simulink model "Formation_no_obs"  (R2023b)
settings: Solver=FixedStepAuto  StartTime=0.0  StopTime=Sim_Time  FixedStep=dt  RelTol=1e-3
values from neighbouring files (symbols this model uses):
  delta_max = 500*pi/180    (= 8.72664625997)    [Run_Formation_no_obs.m]
  psi_r_sat = 10*pi/180    (= 0.174532925199)    [Run_Formation_no_obs.m]
  u0 = 1    [Run_Formation_no_obs.m]
  u_max = 2.5    [Run_Formation_no_obs.m]
  u_min = 0.2    [Run_Formation_no_obs.m]
  Xd = [150; 90]    [Run_Formation_no_obs.m]
  Xob = [750 800; 40 65]    [Run_Formation_no_obs.m]
libraries: slpidlib x3
settings Model: Creator=Behnaz Hadi  LastModifiedBy=ps22aae
settings SolverCC: AlgebraicLoopSolver=TrustRegion
settings DataIOCC: ReturnWorkspaceOutputs=off
settings DebuggingCC: UnconnectedInputMsg=warning  UnconnectedOutputMsg=warning  UnconnectedLineMsg=warning  ArithmeticOperatorsInVariantConditions=warning
settings ModelReferenceCC: EnableRefExpFcnMdlSchedulingChecks=on
settings SFSimCC: CustomCodeUndefinedFunction=UseInterfaceOnly
settings RTWCC: DLArmComputeVersion=19.05

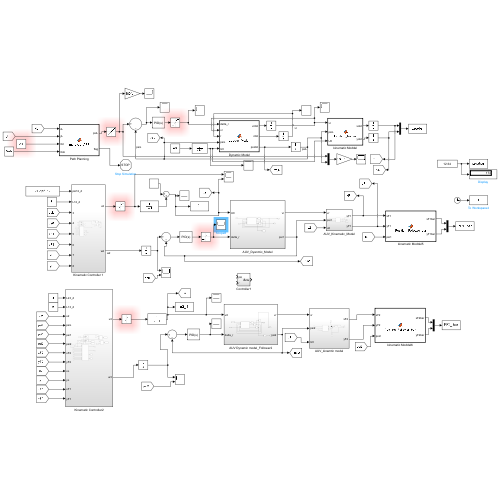
[thumbnail: Simulink's stored preview of the top-level diagram]
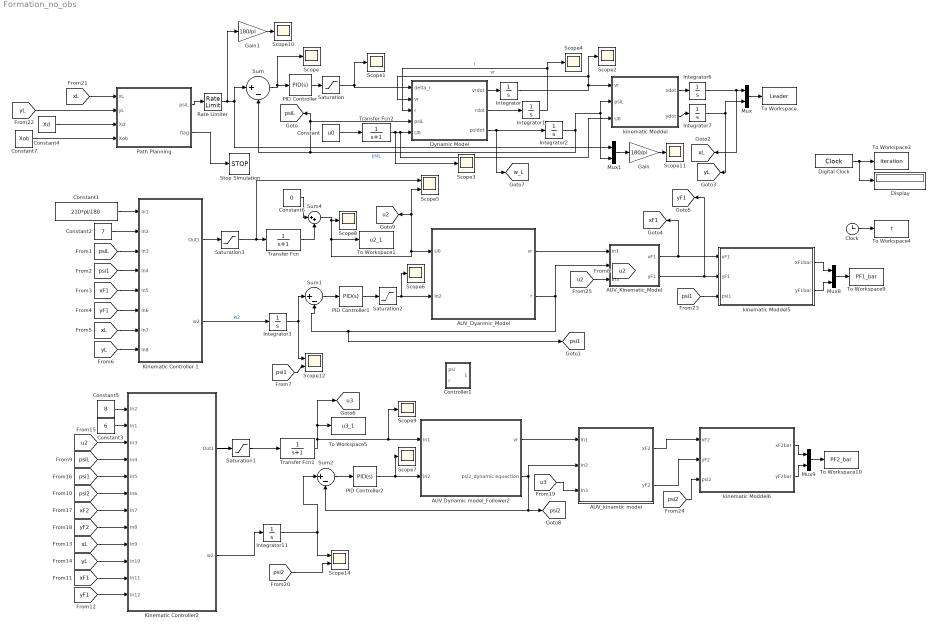
== system Formation_no_obs ==
  AUV Dynamic model_Follower2 : Subsystem
  AUV_Dyanmic_Model : Subsystem
  AUV_Kinematic_Model : Subsystem
  AUV_kinamtic model : Subsystem
  Clock : Clock
  Constant : Constant  Value=u0
  Constant1 : Constant  Value=210*pi/180
  Constant2 : Constant  Value=7
  Constant3 : Constant  Value=6
  Constant4 : Constant  Value=Xd
  Constant5 : Constant  Value=8
  Constant6 : Constant  Value=0
  Constant7 : Constant  Value=Xob
  Controller1 : Subsystem
  Digital Clock : DigitalClock
  Display : Display
  Dynamic Model : MATLAB Function  TreatAsAtomicUnit=on
  Gain : Gain  Gain=180/pi
  Gain1 : Gain  Gain=180/pi
  Integrator{,1,3,11} (4 alike) : Integrator
  Integrator2 : Integrator  InitialCondition=pi/6
  Integrator6 : Integrator  InitialCondition=6
  Integrator7 : Integrator  InitialCondition=4
  Kinematic Controller 1 : Subsystem
  Kinematic Controller2 : Subsystem
  Mux{,1,8..9} (4 alike) : Mux  Inputs=2
  PID Controller : slpidlib/PID Controller  Controller=PID  Form=Ideal  TimeDomain=Continuous-time  UseExternalTs=off  SampleTime=-1  IntegratorMethod=Forward Euler  FilterMethod=Forward Euler  ControllerParametersSource=internal  P=-4.58375331776641  I=0.348826037798542  UseKiTs=off  D=0.667672634240164  N=10.0336095861132  UseFilter=on  TunerSelectOption=Transfer Function Based (PID Tuner App)  InitialConditionSource=internal  InitialConditionForIntegrator=0  InitialConditionForFilter=0  DifferentiatorICPrevScaledInput=0  ExternalReset=none  TrackingMode=off  Kt=1  LimitOutput=off  SatLimitsSource=internal  UpperSaturationLimit=inf  LowerSaturationLimit=-inf  LinearizeAsGain=on  AntiWindupMode=none  Kb=1  LimitIntegrator=off  UpperIntegratorSaturationLimit=inf  LowerIntegratorSaturationLimit=-inf  POutMin=[]  POutMax=[]  IOutMin=[]  IOutMax=[]  DOutMin=[]  DOutMax=[]  NOutMin=[]  NOutMax=[]  SumOutMin=[]  SumOutMax=[]  SaturationOutMin=[]  SaturationOutMax=[]  PParamMin=[]  PParamMax=[]  IParamMin=[]  IParamMax=[]  DParamMin=[]  DParamMax=[]  NParamMin=[]  NParamMax=[]  KbParamMin=[]  KbParamMax=[]  KtParamMin=[]  KtParamMax=[]  KbOutMin=[]  KbOutMax=[]  KtOutMin=[]  KtOutMax=[]  IntegratorOutMin=[]  IntegratorOutMax=[]  FilterOutMin=[]  FilterOutMax=[]  SumI1OutMin=[]  SumI1OutMax=[]  SumI2OutMin=[]  SumI2OutMax=[]  SumI3OutMin=[]  SumI3OutMax=[]  SumI4OutMin=[]  SumI4OutMax=[]  SumDOutMin=[]  SumDOutMax=[]  DifferentiatorOutMin=[]  DifferentiatorOutMax=[]  FilterDiffOutCoefMin=[]  FilterDiffOutCoefMax=[]  ReciprocalOutMin=[]  ReciprocalOutMax=[]  SumDenOutMin=[]  SumDenOutMax=[]  SumNumOutMin=[]  SumNumOutMax=[]  DivideOutMin=[]  DivideOutMax=[]  UdiffTsProdOutMin=[]  UdiffTsProdOutMax=[]  NTsProdOutMin=[]  NTsProdOutMax=[]  UintegralTsProdOutMin=[]  UintegralTsProdOutMax=[]  UngainTsProdOutMin=[]  UngainTsProdOutMax=[]  ClampingZeroOutDataTypeStr=Inherit: Inherit via back propagation  ClampingZeroOutMin=[]  ClampingZeroOutMax=[]  FilterDenConstantOutDataTypeStr=Inherit: Inherit via back propagation  FilterDenConstantOutMin=[]  FilterDenConstantOutMax=[]  PCopyOutDataTypeStr=Inherit: Inherit via back propagation  PCopyOutMin=[]  PCopyOutMax=[]  NCopyOutDataTypeStr=Inherit: Inherit via back propagation  NCopyOutMin=[]  NCopyOutMax=[]  IntegratorContinuousStateAttributes=''  IntegratorStateMustResolveToSignalObject=off  IntegratorRTWStateStorageClass=Auto  FilterContinuousStateAttributes=''  FilterStateMustResolveToSignalObject=off  FilterRTWStateStorageClass=Auto  ParallelPVariant=Passthrough  IdealPVariant=InternalParameters  IVariant=InternalParameters  DVariant=InternalParameters  IntegratorVariant=Continuous  SatVariant=Disabled  AWVariant=Passthrough  PCopyVariant=Disabled  TRVariant=Disabled  FdbkBlocksVariant=Forward  IdealPFdbkVariant=Disabled  SatFdbkVariant=Disabled  DerivativeFilterVariant=ContFilter  NVariant=InternalParameters  NCopyVariant=Disabled  FilterICVariant=InternalICsFilter  IntegratorICVariant=InternalICs  ExternalResetVariant=Disabled  TRSumVariant=Passthrough  SumFdbkVariant=Disabled  SumVariant=Sum_PID  TsampFilterVariant=InternalTs  TsampNgainVariant=Passthrough  TsampIntegralVariant=Disabled_SignalSpec  ExternalSaturationOutDataTypeStr=Inherit: Same as second input
  PID Controller1 : slpidlib/PID Controller  Controller=PID  Form=Ideal  TimeDomain=Continuous-time  UseExternalTs=off  SampleTime=-1  IntegratorMethod=Forward Euler  FilterMethod=Forward Euler  ControllerParametersSource=internal  P=-4001.77706497056  I=5.16468685672513  UseKiTs=off  D=0.0301092952716466  N=1498.86057427308  UseFilter=on  TunerSelectOption=Transfer Function Based (PID Tuner App)  InitialConditionSource=internal  InitialConditionForIntegrator=0  InitialConditionForFilter=0  DifferentiatorICPrevScaledInput=0  ExternalReset=none  TrackingMode=off  Kt=1  LimitOutput=off  SatLimitsSource=internal  UpperSaturationLimit=inf  LowerSaturationLimit=-inf  LinearizeAsGain=on  AntiWindupMode=none  Kb=1  LimitIntegrator=off  UpperIntegratorSaturationLimit=inf  LowerIntegratorSaturationLimit=-inf  POutMin=[]  POutMax=[]  IOutMin=[]  IOutMax=[]  DOutMin=[]  DOutMax=[]  NOutMin=[]  NOutMax=[]  SumOutMin=[]  SumOutMax=[]  SaturationOutMin=[]  SaturationOutMax=[]  PParamMin=[]  PParamMax=[]  IParamMin=[]  IParamMax=[]  DParamMin=[]  DParamMax=[]  NParamMin=[]  NParamMax=[]  KbParamMin=[]  KbParamMax=[]  KtParamMin=[]  KtParamMax=[]  KbOutMin=[]  KbOutMax=[]  KtOutMin=[]  KtOutMax=[]  IntegratorOutMin=[]  IntegratorOutMax=[]  FilterOutMin=[]  FilterOutMax=[]  SumI1OutMin=[]  SumI1OutMax=[]  SumI2OutMin=[]  SumI2OutMax=[]  SumI3OutMin=[]  SumI3OutMax=[]  SumI4OutMin=[]  SumI4OutMax=[]  SumDOutMin=[]  SumDOutMax=[]  DifferentiatorOutMin=[]  DifferentiatorOutMax=[]  FilterDiffOutCoefMin=[]  FilterDiffOutCoefMax=[]  ReciprocalOutMin=[]  ReciprocalOutMax=[]  SumDenOutMin=[]  SumDenOutMax=[]  SumNumOutMin=[]  SumNumOutMax=[]  DivideOutMin=[]  DivideOutMax=[]  UdiffTsProdOutMin=[]  UdiffTsProdOutMax=[]  NTsProdOutMin=[]  NTsProdOutMax=[]  UintegralTsProdOutMin=[]  UintegralTsProdOutMax=[]  UngainTsProdOutMin=[]  UngainTsProdOutMax=[]  ClampingZeroOutDataTypeStr=Inherit: Inherit via back propagation  ClampingZeroOutMin=[]  ClampingZeroOutMax=[]  FilterDenConstantOutDataTypeStr=Inherit: Inherit via back propagation  FilterDenConstantOutMin=[]  FilterDenConstantOutMax=[]  PCopyOutDataTypeStr=Inherit: Inherit via back propagation  PCopyOutMin=[]  PCopyOutMax=[]  NCopyOutDataTypeStr=Inherit: Inherit via back propagation  NCopyOutMin=[]  NCopyOutMax=[]  IntegratorContinuousStateAttributes=''  IntegratorStateMustResolveToSignalObject=off  IntegratorRTWStateStorageClass=Auto  FilterContinuousStateAttributes=''  FilterStateMustResolveToSignalObject=off  FilterRTWStateStorageClass=Auto  ParallelPVariant=Passthrough  IdealPVariant=InternalParameters  IVariant=InternalParameters  DVariant=InternalParameters  IntegratorVariant=Continuous  SatVariant=Disabled  AWVariant=Passthrough  PCopyVariant=Disabled  TRVariant=Disabled  FdbkBlocksVariant=Forward  IdealPFdbkVariant=Disabled  SatFdbkVariant=Disabled  DerivativeFilterVariant=ContFilter  NVariant=InternalParameters  NCopyVariant=Disabled  FilterICVariant=InternalICsFilter  IntegratorICVariant=InternalICs  ExternalResetVariant=Disabled  TRSumVariant=Passthrough  SumFdbkVariant=Disabled  SumVariant=Sum_PID  TsampFilterVariant=InternalTs  TsampNgainVariant=Passthrough  TsampIntegralVariant=Disabled_SignalSpec  ExternalSaturationOutDataTypeStr=Inherit: Same as second input
  PID Controller2 : slpidlib/PID Controller  Controller=PID  Form=Ideal  TimeDomain=Continuous-time  UseExternalTs=off  SampleTime=-1  IntegratorMethod=Forward Euler  FilterMethod=Forward Euler  ControllerParametersSource=internal  P=-22  I=0  UseKiTs=off  D=0.4  N=68.9458315113197  UseFilter=on  TunerSelectOption=Transfer Function Based (PID Tuner App)  InitialConditionSource=internal  InitialConditionForIntegrator=0  InitialConditionForFilter=0  DifferentiatorICPrevScaledInput=0  ExternalReset=none  TrackingMode=off  Kt=1  LimitOutput=off  SatLimitsSource=internal  UpperSaturationLimit=inf  LowerSaturationLimit=-inf  LinearizeAsGain=on  AntiWindupMode=none  Kb=1  LimitIntegrator=off  UpperIntegratorSaturationLimit=inf  LowerIntegratorSaturationLimit=-inf  POutMin=[]  POutMax=[]  IOutMin=[]  IOutMax=[]  DOutMin=[]  DOutMax=[]  NOutMin=[]  NOutMax=[]  SumOutMin=[]  SumOutMax=[]  SaturationOutMin=[]  SaturationOutMax=[]  PParamMin=[]  PParamMax=[]  IParamMin=[]  IParamMax=[]  DParamMin=[]  DParamMax=[]  NParamMin=[]  NParamMax=[]  KbParamMin=[]  KbParamMax=[]  KtParamMin=[]  KtParamMax=[]  KbOutMin=[]  KbOutMax=[]  KtOutMin=[]  KtOutMax=[]  IntegratorOutMin=[]  IntegratorOutMax=[]  FilterOutMin=[]  FilterOutMax=[]  SumI1OutMin=[]  SumI1OutMax=[]  SumI2OutMin=[]  SumI2OutMax=[]  SumI3OutMin=[]  SumI3OutMax=[]  SumI4OutMin=[]  SumI4OutMax=[]  SumDOutMin=[]  SumDOutMax=[]  DifferentiatorOutMin=[]  DifferentiatorOutMax=[]  FilterDiffOutCoefMin=[]  FilterDiffOutCoefMax=[]  ReciprocalOutMin=[]  ReciprocalOutMax=[]  SumDenOutMin=[]  SumDenOutMax=[]  SumNumOutMin=[]  SumNumOutMax=[]  DivideOutMin=[]  DivideOutMax=[]  UdiffTsProdOutMin=[]  UdiffTsProdOutMax=[]  NTsProdOutMin=[]  NTsProdOutMax=[]  UintegralTsProdOutMin=[]  UintegralTsProdOutMax=[]  UngainTsProdOutMin=[]  UngainTsProdOutMax=[]  ClampingZeroOutDataTypeStr=Inherit: Inherit via back propagation  ClampingZeroOutMin=[]  ClampingZeroOutMax=[]  FilterDenConstantOutDataTypeStr=Inherit: Inherit via back propagation  FilterDenConstantOutMin=[]  FilterDenConstantOutMax=[]  PCopyOutDataTypeStr=Inherit: Inherit via back propagation  PCopyOutMin=[]  PCopyOutMax=[]  NCopyOutDataTypeStr=Inherit: Inherit via back propagation  NCopyOutMin=[]  NCopyOutMax=[]  IntegratorContinuousStateAttributes=''  IntegratorStateMustResolveToSignalObject=off  IntegratorRTWStateStorageClass=Auto  FilterContinuousStateAttributes=''  FilterStateMustResolveToSignalObject=off  FilterRTWStateStorageClass=Auto  ParallelPVariant=Passthrough  IdealPVariant=InternalParameters  IVariant=InternalParameters  DVariant=InternalParameters  IntegratorVariant=Continuous  SatVariant=Disabled  AWVariant=Passthrough  PCopyVariant=Disabled  TRVariant=Disabled  FdbkBlocksVariant=Forward  IdealPFdbkVariant=Disabled  SatFdbkVariant=Disabled  DerivativeFilterVariant=ContFilter  NVariant=InternalParameters  NCopyVariant=Disabled  FilterICVariant=InternalICsFilter  IntegratorICVariant=InternalICs  ExternalResetVariant=Disabled  TRSumVariant=Passthrough  SumFdbkVariant=Disabled  SumVariant=Sum_PID  TsampFilterVariant=InternalTs  TsampNgainVariant=Passthrough  TsampIntegralVariant=Disabled_SignalSpec  ExternalSaturationOutDataTypeStr=Inherit: Same as second input
  Path Planning : MATLAB Function  TreatAsAtomicUnit=on
  Rate Limiter : RateLimiter  RisingSlewLimit=psi_r_sat  FallingSlewLimit=-psi_r_sat  SampleTimeMode=inherited
  Saturation : Saturate  UpperLimit=delta_max  LowerLimit=-delta_max
  Saturation1 : Saturate  UpperLimit=u_max  LowerLimit=u_min
  Saturation2 : Saturate  UpperLimit=delta_max  LowerLimit=-delta_max
  Saturation3 : Saturate  UpperLimit=u_max  LowerLimit=u_min
  Scope{,1..4,6..11} (11 alike) : Scope
  Scope12 : Scope  NumInputPorts=2
  Scope14 : Scope  NumInputPorts=2
  Scope5 : Scope  NumInputPorts=2
  Stop Simulation : Stop
  Sum : Sum  Inputs=|+-
  Sum1 : Sum  Inputs=|+-
  Sum2 : Sum  Inputs=|+-
  Sum4 : Sum  Inputs=|++
  To Workspace : ToWorkspace  VariableName=Leader  SampleTime=-1
  To Workspace1 : ToWorkspace  VariableName=u2_1  SampleTime=-1
  To Workspace10 : ToWorkspace  VariableName=PF2_bar  SampleTime=-1
  To Workspace3 : ToWorkspace  VariableName=iteration  SampleTime=-1
  To Workspace4 : ToWorkspace  VariableName=t  SampleTime=-1
  To Workspace5 : ToWorkspace  VariableName=u3_1  SampleTime=-1
  To Workspace9 : ToWorkspace  VariableName=PF1_bar  SampleTime=-1
  Transfer Fcn : TransferFcn  Denominator=[1 1]
  Transfer Fcn1 : TransferFcn  Denominator=[1 1]
  Transfer Fcn2 : TransferFcn  Denominator=[1 1]
  kinematic Moddel : MATLAB Function  TreatAsAtomicUnit=on
  kinematic Moddel5 : MATLAB Function  TreatAsAtomicUnit=on
  kinematic Moddel6 : MATLAB Function  TreatAsAtomicUnit=on
  tag scope: psi1=global, psi2=global, psiL=global, u2=global, u3=global, w_L=global, xF1=global, xL=global, yF1=global, yL=global
  wires:
  [xL] -> Path Planning/1(xL)
  [yL] -> Path Planning/2(yL)
  Path Planning/2(flag) -> Stop Simulation/1
  Path Planning/1(psiL) -> Rate Limiter/1
  kinematic Moddel/1(xdot) -> Integrator6/1
  Integrator6/1 -> [xL], Mux/1
  kinematic Moddel/2(ydot) -> Integrator7/1
  Mux1/1 -> Gain/1
  Integrator1/1 -> Scope4/1, Dynamic Model/3(r)  "r"
  Dynamic Model/1(vrdot) -> Integrator/1
  Saturation/1 -> Dynamic Model/1(delta_r), Scope1/1
  Dynamic Model/3(psidot) -> Integrator2/1, [w_L]
  Integrator2/1 -> Mux1/2, kinematic Moddel/2(psiL), Dynamic Model/4(psiL), [psiL], Sum/2  "psiL"
  Sum/1 -> PID Controller/1, Scope/1
  Integrator7/1 -> [yL], Mux/2
  Integrator/1 -> Dynamic Model/2(vr), Scope2/1, kinematic Moddel/1(vr)  "vr"
  Mux/1 -> To Workspace/1
  Dynamic Model/2(rdot) -> Integrator1/1
  Clock/1 -> To Workspace4/1
  Digital Clock/1 -> Display/1, To Workspace3/1
  Sum1/1 -> PID Controller1/1
  Sum2/1 -> PID Controller2/1
  kinematic Moddel5/1(xF1bar) -> Mux8/1
  kinematic Moddel5/2(yF1bar) -> Mux8/2
  Mux8/1 -> To Workspace9/1
  kinematic Moddel6/2(yF2bar) -> Mux9/2
  kinematic Moddel6/1(xF2bar) -> Mux9/1
  Mux9/1 -> To Workspace10/1
  [psi2] -> kinematic Moddel6/3(psi2)
  Kinematic Controller 1/2(w2) -> Integrator3/1  "w2"
  Constant1/1 -> Kinematic Controller 1/1(In1)
  Constant2/1 -> Kinematic Controller 1/2(In2)
  [psiL] -> Kinematic Controller 1/3(In3)
  [psi1] -> Kinematic Controller 1/4(In4)
  [xF1] -> Kinematic Controller 1/5(In5)
  [yF1] -> Kinematic Controller 1/6(In6)
  [xL] -> Kinematic Controller 1/7(In7)
  [yL] -> Kinematic Controller 1/8(In8)
  AUV_Dyanmic_Model/2(r) -> AUV_Kinematic_Model/2(In2), Sum1/2, [psi1]
  Kinematic Controller 1/1(Out1) -> Saturation3/1
  [psi1] -> Scope12/2
  AUV_Dyanmic_Model/1(vr) -> AUV_Kinematic_Model/1(In1)
  [u2] -> AUV_Kinematic_Model/3(In3)
  AUV_Kinematic_Model/1(xF1) -> [xF1], kinematic Moddel5/1(xF1)
  AUV_Kinematic_Model/2(yF1) -> [yF1], kinematic Moddel5/2(yF1)
  [psi1] -> kinematic Moddel5/3(psi1)
  Kinematic Controller2/2(w2) -> Integrator11/1
  Constant3/1 -> Kinematic Controller2/2(In1)
  [u2] -> Kinematic Controller2/3(In3)
  [psiL] -> Kinematic Controller2/4(In4)
  [psi1] -> Kinematic Controller2/5(In5)
  [psi2] -> Kinematic Controller2/6(In6)
  [xF2] -> Kinematic Controller2/7(In7)
  [yF2] -> Kinematic Controller2/8(In8)
  [xL] -> Kinematic Controller2/9(In9)
  [yL] -> Kinematic Controller2/10(In10)
  [xF1] -> Kinematic Controller2/11(In11)
  [yF1] -> Kinematic Controller2/12(In12)
  Constant5/1 -> Kinematic Controller2/1(In2)
  AUV Dynamic model_Follower2/2(psi2_dynamic equaction) -> AUV_kinamtic model/2(In2), [psi2], Sum2/2
  Kinematic Controller2/1(Out1) -> Saturation1/1
  [psi2] -> Scope14/2
  AUV Dynamic model_Follower2/1(vr) -> AUV_kinamtic model/1(In1)
  [u3] -> AUV_kinamtic model/3(In3)
  AUV_kinamtic model/1(xF2) -> kinematic Moddel6/1(xF2)
  AUV_kinamtic model/2(yF2) -> kinematic Moddel6/2(yF2)
  Integrator11/1 -> Scope14/1, Sum2/1
  Integrator3/1 -> Scope12/1, Sum1/1
  Sum4/1 -> Scope5/2, [u2], AUV_Dyanmic_Model/1(U0), To Workspace1/1, Scope8/1
  Transfer Fcn1/1 -> [u3], To Workspace5/1, Scope9/1, AUV Dynamic model_Follower2/1(In1)
  PID Controller2/1 -> AUV Dynamic model_Follower2/2(In2), Scope7/1
  PID Controller/1 -> Saturation/1
  Rate Limiter/1 -> Gain1/1, Sum/1, Mux1/1
  PID Controller1/1 -> Saturation2/1
  Gain/1 -> Scope11/1
  Gain1/1 -> Scope10/1
  Constant/1 -> Transfer Fcn2/1
  Saturation2/1 -> Scope6/1, AUV_Dyanmic_Model/2(In2)
  Transfer Fcn/1 -> Sum4/2
  Constant6/1 -> Sum4/1
  Constant4/1 -> Path Planning/3(Xd)
  Constant7/1 -> Path Planning/4(Xob)
  Saturation1/1 -> Transfer Fcn1/1
  Saturation3/1 -> Transfer Fcn/1, Scope5/1
  Transfer Fcn2/1 -> Scope3/1, kinematic Moddel/3(U0), Dynamic Model/5(U0)

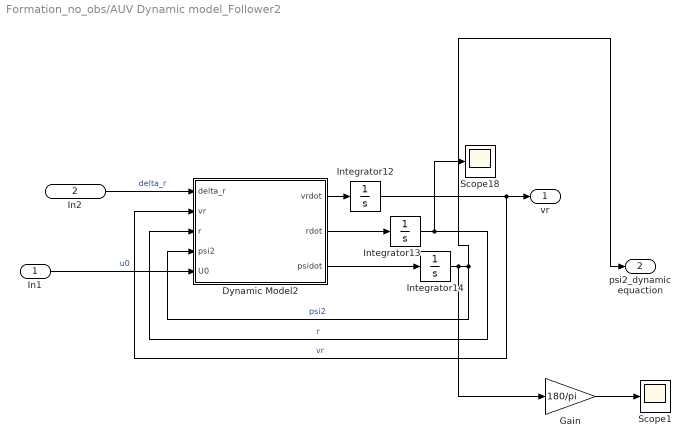
== system Formation_no_obs/AUV Dynamic model_Follower2 ==
  In1 : Inport
  In2 : Inport  Port=2
  Dynamic Model2 : MATLAB Function  TreatAsAtomicUnit=on
  Gain : Gain  Gain=180/pi
  Integrator12 : Integrator
  Integrator13 : Integrator
  Integrator14 : Integrator  InitialCondition=pi/6
  Scope1 : Scope
  Scope18 : Scope
  vr : Outport  VectorParamsAs1DForOutWhenUnconnected=off
  psi2_dynamic equaction : Outport  Port=2  VectorParamsAs1DForOutWhenUnconnected=off
  wires:
  In1/1 -> Dynamic Model2/5(U0)  "u0"
  Dynamic Model2/2(rdot) -> Integrator13/1
  Integrator13/1 -> Scope18/1, Dynamic Model2/3(r)  "r"
  In2/1 -> Dynamic Model2/1(delta_r)  "delta_r"
  Integrator12/1 -> vr/1, Dynamic Model2/2(vr)  "vr"
  Dynamic Model2/3(psidot) -> Integrator14/1
  Dynamic Model2/1(vrdot) -> Integrator12/1
  Integrator14/1 -> Gain/1, psi2_dynamic equaction/1, Dynamic Model2/4(psi2)  "psi2"
  Gain/1 -> Scope1/1

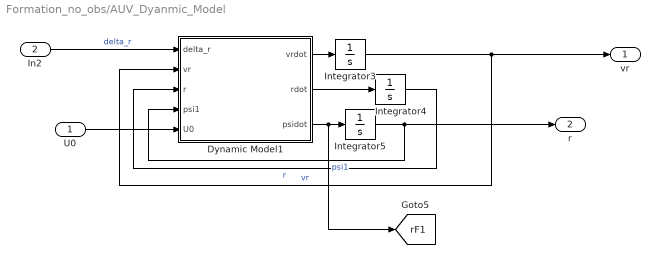
== system Formation_no_obs/AUV_Dyanmic_Model ==
  U0 : Inport
  In2 : Inport  Port=2
  Dynamic Model1 : MATLAB Function  TreatAsAtomicUnit=on
  Integrator3 : Integrator
  Integrator4 : Integrator
  Integrator5 : Integrator
  vr : Outport  VectorParamsAs1DForOutWhenUnconnected=off
  r : Outport  Port=2  VectorParamsAs1DForOutWhenUnconnected=off
  tag scope: rF1=global
  wires:
  Integrator4/1 -> Dynamic Model1/3(r)  "r"
  Dynamic Model1/1(vrdot) -> Integrator3/1
  Dynamic Model1/2(rdot) -> Integrator4/1
  Dynamic Model1/3(psidot) -> [rF1], Integrator5/1
  U0/1 -> Dynamic Model1/5(U0)
  Integrator3/1 -> vr/1, Dynamic Model1/2(vr)  "vr"
  Integrator5/1 -> Dynamic Model1/4(psi1), r/1  "psi1"
  In2/1 -> Dynamic Model1/1(delta_r)  "delta_r"

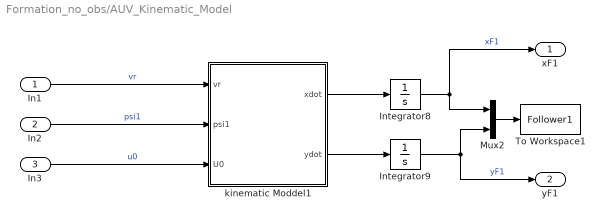
== system Formation_no_obs/AUV_Kinematic_Model ==
  In1 : Inport
  In2 : Inport  Port=2
  In3 : Inport  Port=3
  Integrator8 : Integrator  InitialCondition=7
  Integrator9 : Integrator  InitialCondition=2
  Mux2 : Mux  Inputs=2
  To Workspace1 : ToWorkspace  VariableName=Follower1  SampleTime=-1
  kinematic Moddel1 : MATLAB Function  TreatAsAtomicUnit=on
  xF1 : Outport  VectorParamsAs1DForOutWhenUnconnected=off
  yF1 : Outport  Port=2  VectorParamsAs1DForOutWhenUnconnected=off
  wires:
  kinematic Moddel1/2(ydot) -> Integrator9/1
  kinematic Moddel1/1(xdot) -> Integrator8/1
  Mux2/1 -> To Workspace1/1
  Integrator9/1 -> yF1/1, Mux2/2  "yF1"
  Integrator8/1 -> Mux2/1, xF1/1  "xF1"
  In1/1 -> kinematic Moddel1/1(vr)  "vr"
  In2/1 -> kinematic Moddel1/2(psi1)  "psi1"
  In3/1 -> kinematic Moddel1/3(U0)  "u0"

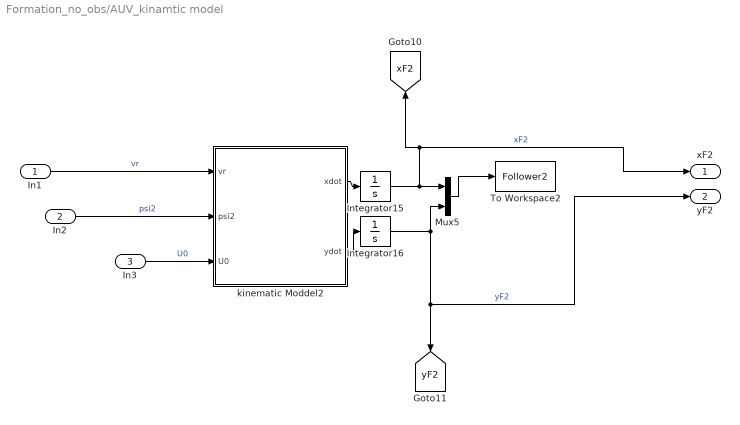
== system Formation_no_obs/AUV_kinamtic model ==
  In1 : Inport
  In2 : Inport  Port=2
  In3 : Inport  Port=3
  Integrator15 : Integrator  InitialCondition=2
  Integrator16 : Integrator  InitialCondition=1
  Mux5 : Mux  Inputs=2
  To Workspace2 : ToWorkspace  VariableName=Follower2  SampleTime=-1
  kinematic Moddel2 : MATLAB Function  TreatAsAtomicUnit=on
  xF2 : Outport  VectorParamsAs1DForOutWhenUnconnected=off
  yF2 : Outport  Port=2  VectorParamsAs1DForOutWhenUnconnected=off
  tag scope: xF2=global, yF2=global
  wires:
  Integrator15/1 -> xF2/1, [xF2], Mux5/1  "xF2"
  Integrator16/1 -> Mux5/2, yF2/1, [yF2]  "yF2"
  kinematic Moddel2/2(ydot) -> Integrator16/1
  In1/1 -> kinematic Moddel2/1(vr)  "vr"
  kinematic Moddel2/1(xdot) -> Integrator15/1
  Mux5/1 -> To Workspace2/1
  In3/1 -> kinematic Moddel2/3(U0)  "U0"
  In2/1 -> kinematic Moddel2/2(psi2)  "psi2"

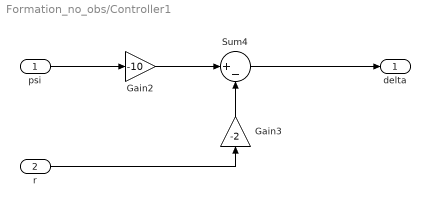
== system Formation_no_obs/Controller1 ==
  psi : Inport
  r : Inport  Port=2
  Gain2 : Gain  Gain=-10
  Gain3 : Gain  Gain=-2
  Sum4 : Sum  Inputs=|+-
  delta : Outport
  wires:
  Gain2/1 -> Sum4/1
  Gain3/1 -> Sum4/2
  psi/1 -> Gain2/1
  Sum4/1 -> delta/1
  r/1 -> Gain3/1

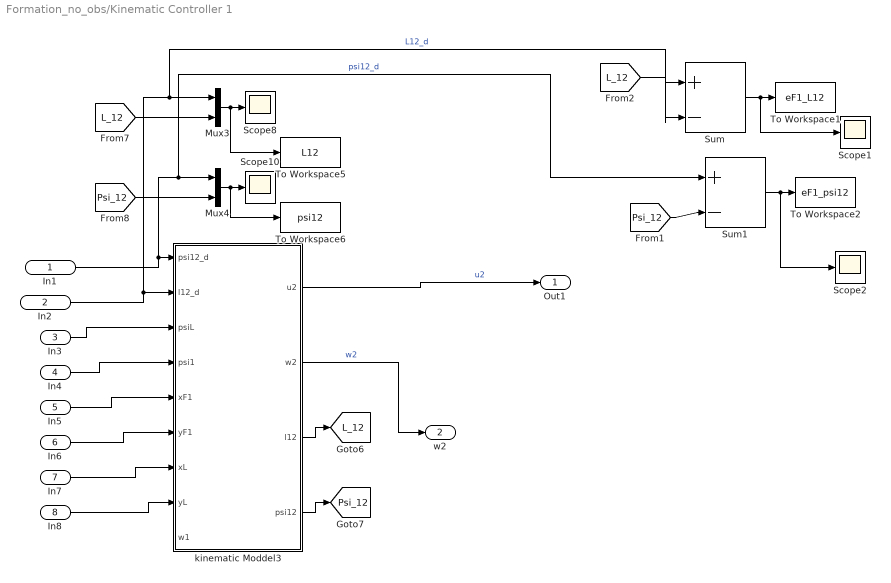
== system Formation_no_obs/Kinematic Controller 1 ==
  In1 : Inport
  In2 : Inport  Port=2
  In3 : Inport  Port=3
  In4 : Inport  Port=4
  In5 : Inport  Port=5
  In6 : Inport  Port=6
  In7 : Inport  Port=7
  In8 : Inport  Port=8
  Mux3 : Mux  Inputs=2
  Mux4 : Mux  Inputs=2
  Scope{1..2,8,10} (4 alike) : Scope
  Sum : Sum  Inputs=+|-
  Sum1 : Sum  Inputs=+|-
  To Workspace1 : ToWorkspace  VariableName=eF1_L12  SampleTime=-1
  To Workspace2 : ToWorkspace  VariableName=eF1_psi12  SampleTime=-1
  To Workspace5 : ToWorkspace  VariableName=L12  SampleTime=-1
  To Workspace6 : ToWorkspace  VariableName=psi12  SampleTime=-1
  kinematic Moddel3 : MATLAB Function  TreatAsAtomicUnit=on
  Out1 : Outport  VectorParamsAs1DForOutWhenUnconnected=off
  w2 : Outport  Port=2  VectorParamsAs1DForOutWhenUnconnected=off
  tag scope: L_12=global, Psi_12=global
  wires:
  Mux3/1 -> To Workspace5/1, Scope8/1
  [Psi_12] -> Mux4/2
  [L_12] -> Mux3/2
  In8/1 -> kinematic Moddel3/8(yL)
  Mux4/1 -> To Workspace6/1, Scope10/1
  kinematic Moddel3/4(psi12) -> [Psi_12]
  In3/1 -> kinematic Moddel3/3(psiL)
  kinematic Moddel3/3(l12) -> [L_12]
  kinematic Moddel3/2(w2) -> w2/1  "w2"
  In4/1 -> kinematic Moddel3/4(psi1)
  In5/1 -> kinematic Moddel3/5(xF1)
  In6/1 -> kinematic Moddel3/6(yF1)
  In7/1 -> kinematic Moddel3/7(xL)
  kinematic Moddel3/1(u2) -> Out1/1  "u2"
  In2/1 -> Sum/1, Mux3/1, kinematic Moddel3/2(l12_d)  "L12_d"
  In1/1 -> Sum1/1, Mux4/1, kinematic Moddel3/1(psi12_d)  "psi12_d"
  [Psi_12] -> Sum1/2
  Sum1/1 -> Scope2/1, To Workspace2/1
  Sum/1 -> Scope1/1, To Workspace1/1
  [L_12] -> Sum/2

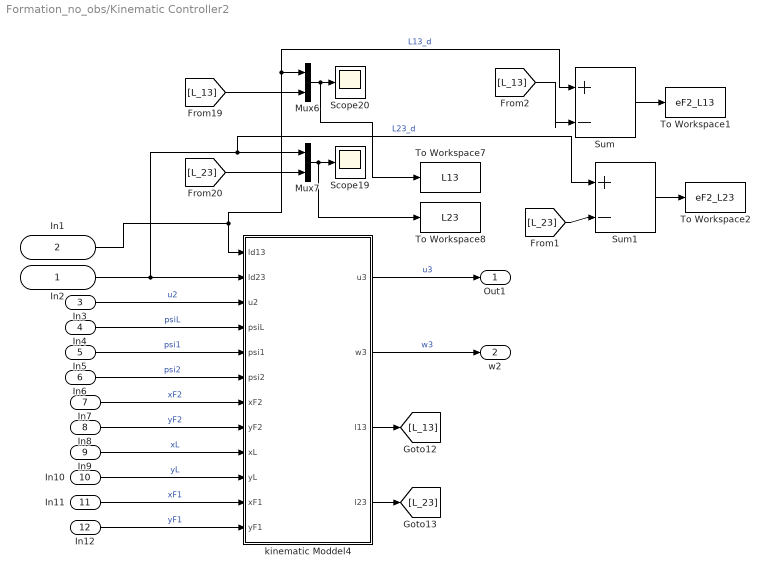
== system Formation_no_obs/Kinematic Controller2 ==
  In2 : Inport
  In1 : Inport  Port=2
  In3 : Inport  Port=3
  In4 : Inport  Port=4
  In5 : Inport  Port=5
  In6 : Inport  Port=6
  In7 : Inport  Port=7
  In8 : Inport  Port=8
  In9 : Inport  Port=9
  In10 : Inport  Port=10
  In11 : Inport  Port=11
  In12 : Inport  Port=12
  Mux6 : Mux  Inputs=2
  Mux7 : Mux  Inputs=2
  Scope19 : Scope
  Scope20 : Scope
  Sum : Sum  Inputs=+|-
  Sum1 : Sum  Inputs=+|-
  To Workspace1 : ToWorkspace  VariableName=eF2_L13  SampleTime=-1
  To Workspace2 : ToWorkspace  VariableName=eF2_L23  SampleTime=-1
  To Workspace7 : ToWorkspace  VariableName=L13  SampleTime=-1
  To Workspace8 : ToWorkspace  VariableName=L23  SampleTime=-1
  kinematic Moddel4 : MATLAB Function  TreatAsAtomicUnit=on
  Out1 : Outport  VectorParamsAs1DForOutWhenUnconnected=off
  w2 : Outport  Port=2  VectorParamsAs1DForOutWhenUnconnected=off
  wires:
  In8/1 -> kinematic Moddel4/8(yF2)  "yF2"
  In6/1 -> kinematic Moddel4/6(psi2)  "psi2"
  kinematic Moddel4/4(l23) -> [L_23]
  In12/1 -> kinematic Moddel4/12(yF1)  "yF1"
  In1/1 -> kinematic Moddel4/1(ld13), Sum/1, Mux6/1  "L13_d"
  [L_23] -> Mux7/2
  Mux7/1 -> To Workspace8/1, Scope19/1
  Mux6/1 -> To Workspace7/1, Scope20/1
  [L_13] -> Mux6/2
  kinematic Moddel4/3(l13) -> [L_13]
  In4/1 -> kinematic Moddel4/4(psiL)  "psiL"
  In10/1 -> kinematic Moddel4/10(yL)  "yL"
  kinematic Moddel4/1(u3) -> Out1/1  "u3"
  In7/1 -> kinematic Moddel4/7(xF2)  "xF2"
  In3/1 -> kinematic Moddel4/3(u2)  "u2"
  kinematic Moddel4/2(w3) -> w2/1  "w3"
  In11/1 -> kinematic Moddel4/11(xF1)  "xF1"
  In5/1 -> kinematic Moddel4/5(psi1)  "psi1"
  In9/1 -> kinematic Moddel4/9(xL)  "xL"
  [L_13] -> Sum/2
  Sum/1 -> To Workspace1/1
  Sum1/1 -> To Workspace2/1
  In2/1 -> kinematic Moddel4/2(ld23), Mux7/1, Sum1/1  "L23_d"
  [L_23] -> Sum1/2

== matlab function Formation_no_obs/AUV_kinamtic model/kinematic Moddel2 ==
  data: vr input; psi2 input; xdot output; ydot output; U0 input
function [xdot,ydot] = Position_Follower(vr,psi2,U0)
% global U0
% U0 = 1.3;
% Ucx =0.2; Ucy =0.2; 
Ucx =0.0; Ucy =0.0; 


% x_dot = U0*cos(sa) - vr*sin(sa)+Ucx;
% y_dot = U0*sin(sa) + vr*cos(sa)+Ucy;
xdot  = U0*cos(psi2) - vr*sin(psi2)+ Ucx ;  %x_dot
ydot  = U0*sin(psi2) + vr*cos(psi2)+ Ucy ;  %y_dot

end

== matlab function Formation_no_obs/Kinematic Controller2/kinematic Moddel4 ==
  data: ld13 input; ld23 input; u2 input; psiL input; psi1 input; psi2 input; u3 output; w3 output; xF2 input; yF2 input; xL input; yL input; xF1 input; yF1 input; l13 output; l23 output
function [u3, w3, l13, l23] = Desai_Controller_TwoNeighbors(ld13, ld23, u2, psiL, psi1, psi2, xF2, yF2, xL, yL, xF1, yF1)
    % Parameters
    u1 = 1.0; d = 0.16;
    alpha1 = 0.2; alpha2 = 0.2;

    % Virtual target point for agent 3 (distance d ahead of follower 2)
    x3b = xF2 + d * cos(psi2);
    y3b = yF2 + d * sin(psi2);

    % psi13: angle from agent L to 3bar
    atan13 = atan2(y3b - yL, x3b - xL);
    if atan13 < 0
        psi13 = 2 * pi + atan13 - psiL;
    else
        psi13 = atan13 - psiL;
    end

    % psi23: angle from agent 1 to 3bar
    atan23 = atan2(y3b - yF1, x3b - xF1);
    if atan23 < 0
        psi23 = 2 * pi + atan23 - psi1;
    else
        psi23 = atan23 - psi1;
    end

    % Inter-agent distances
    l13 = sqrt((xL - x3b)^2 + (yL - y3b)^2);
    l23 = sqrt((xF1 - x3b)^2 + (yF1 - y3b)^2);

    % Heading errors
    gamma1 = psiL + psi13 - psi2;
    gamma2 = psi1 + psi23 - psi2;

    % Wrap angles
    gamma1 = atan2(sin(gamma1), cos(gamma1));
    gamma2 = atan2(sin(gamma2), cos(gamma2));

    % Angular velocity w3
    w3 = (1 / (d * sin(gamma1 - gamma2))) * ...
         ( alpha1 * (ld13 - l13) * cos(gamma2) + u1 * cos(psi13) * cos(gamma2) ...
         - alpha2 * (ld23 - l23) * cos(gamma1) - u2 * cos(psi23) * cos(gamma1) );

    % Linear velocity u3
    u3 = (alpha1 * (ld13 - l13) + u1 * cos(psi13) - d * w3 * sin(gamma1)) / cos(gamma1);
end

== matlab function Formation_no_obs/Path Planning ==
  data: xL input; psiL output; yL input; flag output; Xd input; Xob input
%%%%%%%%%%%%%%% The Basid Method in the book, uncomment if needed %%%%%%%%%
%%%%%%%%%%%%%%%%%%%%%%%%%%%%%%%%%%%%%%%%%%%%%%%%%%%%%%%%%%%%%%%%%%%%%%%%%%%
% function [psiL, flag] = improved_APF(xL, yL, Xd, Xob)
%     % Parameters
%     K_att = 1.0;       % Attractive gain
%     K_rep = 100;         % Repulsive gain
%     rho_0 = 15;        % Repulsion influence range
%     R = 8;             % Obstacle radius
%     flag = 0;          % Goal reached flag
% 
%     % Positions
%     r = [xL; yL];      % Current position
%     rd = Xd;           % Goal position
% 
%     % Attractive force
%     Fatt = -K_att * (r - rd);
% 
%     % Repulsive force
%     Frep = [0; 0];
%     for i = 1:2
%         rob = Xob(:, i);
%         rho = norm(r - rob) - R;
%         if rho <= rho_0
%             diff = r - rob;
%             Frep = Frep + K_rep * (1/rho - 1/rho_0) * (diff / rho^3);
%         end
%     end
% 
%     % Total force and heading
%     F_total = Fatt + Frep;
%     psiL = atan2(F_total(2), F_total(1));
% 
%     % Goal check
%     if norm(rd - r) <= 0.01
%         flag = 1;
%     end
% end

%%%%%%%%%%%%%%% The Improved version from [1], comment if needed %%%%%%%%%%
%% Ge and Cui 2000] Ge, S. S. and Cui, Y. J. (2000). New potential ...
% functions for mobile robot path planning. IEEE Transactions on ...
% robotics and automation[1]
%%%%%%%%%%%%%%%%%%%%%%%%%%%%%%%%%%%%%%%%%%%%%%%%%%%%%%%%%%%%%%%%%%%%%%%%%%%
function [psiL, flag] = improved_APF(xL, yL, Xd, Xob)
    % Parameters
    kp = 1.5;         % Attractive gain
    p0 = 15;          % Repulsion range
    m = 5;           % Repulsion scaling (reduced for smoother psi)
    R = 5;            % Obstacle radius
    N = 2;            % Nonlinearity
    flag = 0;         % Goal reached flag

    % Positions
    XL = [xL; yL];            % Current position

    % Attraction force
    Rat = norm(Xd - XL);
    dir_goal = Xd - XL;
    alpha = atan2(dir_goal(2), dir_goal(1));
    Fatt = kp * Rat * [cos(alpha); sin(alpha)];

    % Repulsion force (sum over both obstacles)
    Frep = [0; 0];
    for i = 1:2
        obs = Xob(:, i);
        Rrep = norm(obs - XL) - R;
        if Rrep <= p0
            F1 = ((1/Rrep) - (1/p0)) * (-(Rat^N) / (Rrep^2));
            F2 = ((1/Rrep - 1/p0)^2) * (Rat^(N - 1));
            Frep_mag = m * F1 + (N/2) * m * F2;
            dir_obs = obs - XL;
            beta = atan2(dir_obs(2), dir_obs(1));
            Frep = Frep + Frep_mag * [cos(beta); sin(beta)];
        end
    end

    % Total force and heading
    F_total = Fatt + Frep;
    psiL = atan2(F_total(2), F_total(1));

    % Goal check
    if norm(Xd - XL) <= 0.01
        flag = 1;
    end
end

== matlab function Formation_no_obs/kinematic Moddel5 ==
  data: xF1 input; yF1 input; xF1bar output; yF1bar output; psi1 input
function [xF1bar,yF1bar] = Position_Follower_bar(xF1,yF1,psi1)
d = 0.16;
xF1bar = xF1+d*cos(psi1);
yF1bar = yF1+d*sin(psi1);

end

== matlab function Formation_no_obs/kinematic Moddel6 ==
  data: xF2 input; yF2 input; xF2bar output; yF2bar output; psi2 input
function [xF2bar,yF2bar] = Position_Follower_bar(xF2,yF2,psi2)
d = 0.16;
xF2bar = xF2+d*cos(psi2);
yF2bar = yF2+d*sin(psi2);

end

== matlab function Formation_no_obs/kinematic Moddel ==
  data: vr input; psiL input; xdot output; ydot output; U0 input
function [xdot,ydot] = Position_leader(vr,psiL,U0)
% global U0

% Ucx =0.2; Ucy =0.2; 
Ucx =0.0; Ucy =0.0; 


% x_dot = U0*cos(sa) - vr*sin(sa)+Ucx;
% y_dot = U0*sin(sa) + vr*cos(sa)+Ucy;
xdot  = U0*cos(psiL) - vr*sin(psiL)+ Ucx ;  %x_dot
ydot  = U0*sin(psiL) + vr*cos(psiL)+ Ucy ;  %y_dot

end

== matlab function Formation_no_obs/Dynamic Model ==
  data: delta_r input; vrdot output; vr input; r input; psiL input; rdot output; psidot output; U0 input
function [vrdot,rdot,psidot] = Leader_Model(delta_r,vr,r,psiL,U0)
% global U0
%U0 =1.0;
m = 30.48;        %kg
Y_vrdot = -35.5;  %kg
Y_rdot = 1.93;    %kg/rad
Y_vr = -66.6;
Y_r = 2.2;        % kgm/s
N_vrdot = 1.93;   % kgm
N_rdot = -4.88;   % kgm2/rad
N_vr = -4.47;     % kgm/s
N_r = -6.87;      % kgm2/s
N_delta = -34.6/3.5;
Y_delta = 50.6/3.5;
Izz = 3.45;       % kgm2/rad 
x_state = [vr;r;psiL];


A =inv([m-Y_vrdot -Y_rdot  0;...
       -N_vrdot Izz-N_rdot 0; ...
        0          0       1]);
B=[Y_vr Y_r-m*U0 0;...
   N_vr   N_r    0;...
    0     1      0];
C=A*B;
D=A*[Y_delta;N_delta;0];

states_vector = A*B*x_state + A*[Y_delta;N_delta;0]*delta_r;
  
vrdot = states_vector(1); rdot = states_vector(2);
psidot = states_vector(3);
%     vrdot  = C(1,1)*x_state(1)+ C(1,2)*x_state(2)+D(1)*delta_r ;  %vr_dot
%     rdot  =  C(2,1)*x_state(1)+ C(2,2)*x_state(2)+D(2)*delta_r ;  %r_dot
%     sadot  = x_state(2) ;  %sa_dot
%     xx(4) = xx(3)*180/pi;
%     
% 
%     if xx(3)> pi
%         xx(3)= xx(3)-2*pi;
%     end
%     if xx(3) < -pi
%         xx(3)= xx(3)+2*pi;
%     end    
end

== matlab function Formation_no_obs/AUV_Dyanmic_Model/Dynamic Model1 ==
  data: delta_r input; vrdot output; vr input; r input; psi1 input; rdot output; psidot output; U0 input
function [vrdot,rdot,psidot] = Follower_Model(delta_r,vr,r,psi1,U0)
% global U0
% U0 =1.3;
m = 30.48;        %kg
Y_vrdot = -35.5;  %kg
Y_rdot = 1.93;    %kg/rad
Y_vr = -66.6;
Y_r = 2.2;        % kgm/s
N_vrdot = 1.93;   % kgm
N_rdot = -4.88;   % kgm2/rad
N_vr = -4.47;     % kgm/s
N_r = -6.87;      % kgm2/s
N_delta = -34.6/3.5;
Y_delta = 50.6/3.5;
Izz = 3.45;       % kgm2/rad 
x_state = [vr;r;psi1];
% xdot_state = inv([m-Y_vrdot -Y_rdot 0; -N_vrdot Izz-N_rdot 0; 0 0 1])*...
%                  [Y_vr Y_r-m*U0 0;N_vr N_r 0; 0 1 0]*x_state+...
%              inv([m-Y_vrdot -Y_rdot 0; -N_vrdot Izz-N_rdot 0; 0 0 1])*[Y_delta;N_delta;0]*delta_r;
A =inv([m-Y_vrdot -Y_rdot  0;...
       -N_vrdot Izz-N_rdot 0; ...
        0          0       1]);
B=[Y_vr Y_r-m*U0 0;...
   N_vr   N_r    0;...
    0     1      0];
C=A*B;
D=A*[Y_delta;N_delta;0];

states_vector = A*B*x_state + A*[Y_delta;N_delta;0]*delta_r;
  
vrdot = states_vector(1); rdot = states_vector(2);
psidot = states_vector(3);
%     vrdot  = C(1,1)*x_state(1)+ C(1,2)*x_state(2)+D(1)*delta_r ;  %vr_dot
%     rdot  =  C(2,1)*x_state(1)+ C(2,2)*x_state(2)+D(2)*delta_r ;  %r_dot
%     sadot  = x_state(2) ;  %sa_dot
%     xx(4) = xx(3)*180/pi;
%     
% 
%     if xx(3)> pi
%         xx(3)= xx(3)-2*pi;
%     end
%     if xx(3) < -pi
%         xx(3)= xx(3)+2*pi;
%     end    
end

== matlab function Formation_no_obs/AUV_Kinematic_Model/kinematic Moddel1 ==
  data: vr input; psi1 input; xdot output; ydot output; U0 input
function [xdot,ydot] = Position_Follower(vr,psi1,U0)
% global U0
% U0 = 1.3;
% Ucx =0.2; Ucy =0.2; 
Ucx =0.0; Ucy =0.0; 


% x_dot = U0*cos(sa) - vr*sin(sa)+Ucx;
% y_dot = U0*sin(sa) + vr*cos(sa)+Ucy;
xdot  = U0*cos(psi1) - vr*sin(psi1)+ Ucx ;  %x_dot
ydot  = U0*sin(psi1) + vr*cos(psi1)+ Ucy ;  %y_dot

end

== matlab function Formation_no_obs/AUV Dynamic model_Follower2/Dynamic Model2 ==
  data: delta_r input; vrdot output; vr input; r input; psi2 input; rdot output; psidot output; U0 input
function [vrdot,rdot,psidot] = Follower_Model(delta_r,vr,r,psi2,U0)
% global U0
% U0 =1.3;
m = 30.48;        %kg
Y_vrdot = -35.5;  %kg
Y_rdot = 1.93;    %kg/rad
Y_vr = -66.6;
Y_r = 2.2;        % kgm/s
N_vrdot = 1.93;   % kgm
N_rdot = -4.88;   % kgm2/rad
N_vr = -4.47;     % kgm/s
N_r = -6.87;      % kgm2/s
N_delta = -34.6/3.5;
Y_delta = 50.6/3.5;
Izz = 3.45;       % kgm2/rad 
x_state = [vr;r;psi2];
% xdot_state = inv([m-Y_vrdot -Y_rdot 0; -N_vrdot Izz-N_rdot 0; 0 0 1])*...
%                  [Y_vr Y_r-m*U0 0;N_vr N_r 0; 0 1 0]*x_state+...
%              inv([m-Y_vrdot -Y_rdot 0; -N_vrdot Izz-N_rdot 0; 0 0 1])*[Y_delta;N_delta;0]*delta_r;
A =inv([m-Y_vrdot -Y_rdot  0;...
       -N_vrdot Izz-N_rdot 0; ...
        0          0       1]);
B=[Y_vr Y_r-m*U0 0;...
   N_vr   N_r    0;...
    0     1      0];
C=A*B;
D=A*[Y_delta;N_delta;0];

states_vector = A*B*x_state + A*[Y_delta;N_delta;0]*delta_r;
  
vrdot = states_vector(1); rdot = states_vector(2);
psidot = states_vector(3);
%     vrdot  = C(1,1)*x_state(1)+ C(1,2)*x_state(2)+D(1)*delta_r ;  %vr_dot
%     rdot  =  C(2,1)*x_state(1)+ C(2,2)*x_state(2)+D(2)*delta_r ;  %r_dot
%     sadot  = x_state(2) ;  %sa_dot
%     xx(4) = xx(3)*180/pi;
%     
% 
%     if xx(3)> pi
%         xx(3)= xx(3)-2*pi;
%     end
%     if xx(3) < -pi
%         xx(3)= xx(3)+2*pi;
%     end    
end

== matlab function Formation_no_obs/Kinematic Controller 1/kinematic Moddel3 ==
  data: psi12_d input; l12_d input; u2 output; w2 output; psiL input; psi1 input; xF1 input; yF1 input; xL input; yL input; l12 output; psi12 output; w1 input
function [u2, w2, l12, psi12] = Desai_Controller(psi12_d, l12_d, psiL, psi1, xF1, yF1, xL, yL, w1)
    % Parameters
    alpha1 = 0.1; alpha2 = 0.1;
    u1 = 1.0; d = 0.16;

    % Follower virtual point (at distance d in heading psi1)
    x2b = xF1 + d * cos(psi1);
    y2b = yF1 + d * sin(psi1);

    % Relative angle psi12 (from leader to virtual point)
    atan12 = atan2(y2b - yL, x2b - xL);
    if atan12 < 0
        psi12 = 2 * pi + atan12 - psiL;
    else
        psi12 = atan12 - psiL;
    end

    % Inter-agent distance
    l12 = sqrt((xL - x2b)^2 + (yL - y2b)^2);

    % Gamma1: total heading error
    gamma1 = psiL + psi12 - psi1;
    gamma1 = atan2(sin(gamma1), cos(gamma1));  % wrap

    % Intermediate control
    rho12 = (alpha1 * (l12_d - l12) + u1 * cos(psi12)) / cos(gamma1);

    % Angular velocity
    w2 = (cos(gamma1)/d) * ( ...
            alpha2 * l12 * (psi12_d - psi12) ...
          - u1 * sin(psi12) ...
          + l12 * w1 ...
          + rho12 * sin(gamma1) );

    % Linear velocity
    u2 = rho12 - d * w2 * tan(gamma1);
end
